simulink model "MRACDevastator"  (R2019a)
settings: Solver=VariableStepAuto  StartTime=0.0  StopTime=10.0  RelTol=1e-3
settings Model: Creator=iris  LastModifiedBy=iris
settings DebuggingCC: SFMachineParentedDataDiag=error

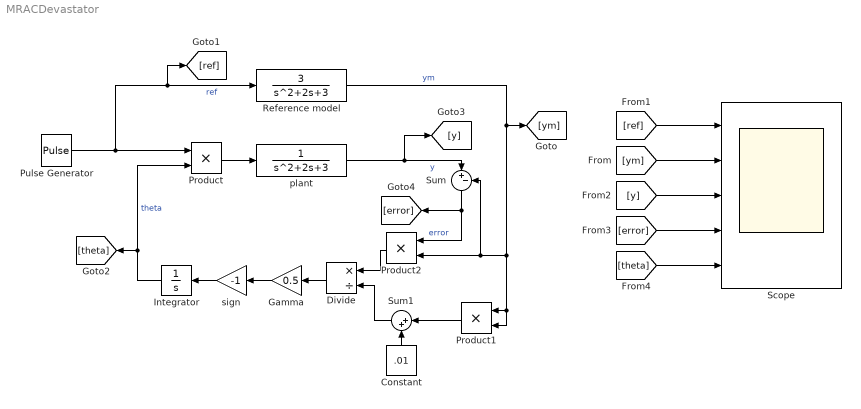
== system MRACDevastator ==
  Constant : Constant  Value=.01
  Divide : Product  Inputs=*/
  Gamma : Gain  Gain=0.5
  Integrator : Integrator
  Product : Product
  Product1 : Product
  Product2 : Product  Inputs=**
  Pulse Generator : DiscretePulseGenerator  PulseType=Time based  PulseWidth=30
  Reference model : TransferFcn  Numerator=[3]  Denominator=[1 2 3]
  Scope : Scope  NumInputPorts=5
  Sum : Sum  Inputs=|+-
  Sum1 : Sum  Inputs=|++
  plant : TransferFcn  Denominator=[1 2 3]
  sign : Gain  Gain=-1
  wires:
  Product/1 -> plant/1
  Pulse Generator/1 -> Product/1, [ref], Reference model/1  "ref"
  plant/1 -> [y], Sum/1  "y"
  Reference model/1 -> [ym], Product2/2, Sum/2, Product1/2, Product1/1  "ym"
  Product1/1 -> Sum1/1
  Sum1/1 -> Divide/2
  Constant/1 -> Sum1/2
  Sum/1 -> [error], Product2/1  "error"
  Product2/1 -> Divide/1
  Divide/1 -> Gamma/1
  Gamma/1 -> sign/1
  Integrator/1 -> [theta], Product/2  "theta"
  sign/1 -> Integrator/1
  [ym] -> Scope/2
  [ref] -> Scope/1
  [y] -> Scope/3
  [error] -> Scope/4
  [theta] -> Scope/5
